simulink model "DL_wKoopman_SimulinkModel"  (R2020b)
settings: Solver=VariableStepAuto  StartTime=0.0  StopTime=10.0  RelTol=1e-3
values from neighbouring files (symbols this model uses):
  B = 0.00732    [DCMotor_Shifted.m]
  C2_new = C2_lift    [DL_wKoopman.m]
  IC_augmented = [x0' zeros(1,Nlift+Nrbf)]    [DL_wKoopman.m]
  IC_original = [x0' zeros(1,Nrbf)]    [DL_wKoopman.m]
  J = 0.00441    [DCMotor_Shifted.m]
  K = dlqr(A_new,B2_new,Q,R)    [DL_wKoopman.m]
  km = 0.253    [DCMotor_Shifted.m]
  La = 0.314    [DCMotor_Shifted.m]
  Ra = 12.345    [DCMotor_Shifted.m]
  sysKF = ss(A_new-Kf*C2_new,[B2_new Kf],eye(Nlift),0*[B2_new Kf])    [DL_wKoopman.m]
  taul = 1.47    [DCMotor_Shifted.m]
  ua = 60    [DCMotor_Shifted.m]
  x0 = [5;30]    [DL_wKoopman.m]
undefined symbols (not defined in the file or in its folder): K_hinf_aug
libraries: simulink x1
settings Model: Creator=anujpal  LastModifiedBy=anujpal

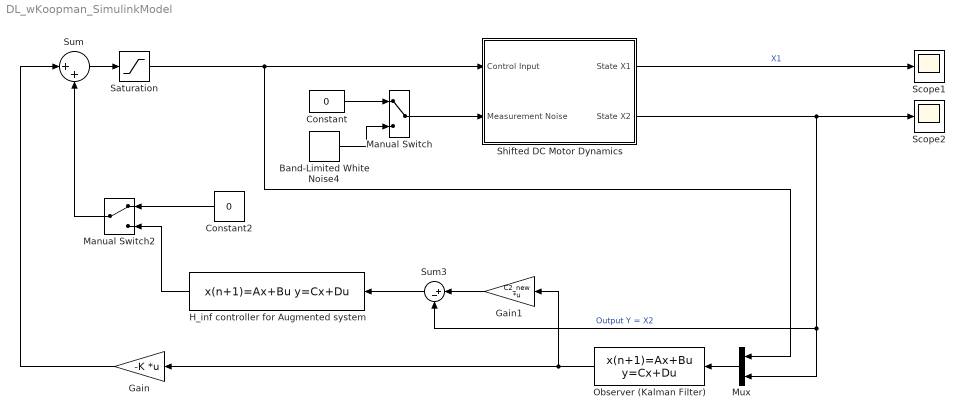
== system DL_wKoopman_SimulinkModel ==
  Band-Limited White Noise4 : simulink/Sources/Band-Limited White Noise  Cov=1  Ts=0.01  seed=245
  Constant : Constant  Value=0
  Constant2 : Constant  Value=0
  Gain : Gain  Gain=-K  Multiplication=Matrix(K*u) (u vector)
  Gain1 : Gain  Gain=C2_new  Multiplication=Matrix(K*u) (u vector)
  H_inf controller for Augmented system : DiscreteStateSpace  A=K_hinf_aug.A  B=K_hinf_aug.B  C=K_hinf_aug.C  D=K_hinf_aug.D  InitialCondition=IC_augmented  SampleTime=-1
  Manual Switch : ManualSwitch
  Manual Switch2 : ManualSwitch
  Mux : Mux  Inputs=2
  Observer (Kalman Filter) : DiscreteStateSpace  A=sysKF.A  B=sysKF.B  C=sysKF.C  D=sysKF.D  InitialCondition=IC_original  SampleTime=-1
  Saturation : Saturate  UpperLimit=4  LowerLimit=-4
  Scope1 : Scope
  Scope2 : Scope
  Shifted DC Motor Dynamics : Subsystem
  Sum : Sum  Inputs=|++
  Sum3 : Sum  Inputs=|+-
  wires:
  Shifted DC Motor Dynamics/2(State X2) -> Scope2/1, Mux/2, Sum3/2  "Output Y = X2"
  Manual Switch/1 -> Shifted DC Motor Dynamics/2(Measurement Noise)
  Shifted DC Motor Dynamics/1(State X1) -> Scope1/1  "X1"
  Sum3/1 -> H_inf controller for Augmented system/1
  Observer (Kalman Filter)/1 -> Gain/1, Gain1/1
  Sum/1 -> Saturation/1
  Constant/1 -> Manual Switch/1
  Mux/1 -> Observer (Kalman Filter)/1
  Constant2/1 -> Manual Switch2/1
  Manual Switch2/1 -> Sum/2
  H_inf controller for Augmented system/1 -> Manual Switch2/2
  Gain/1 -> Sum/1
  Band-Limited White Noise4/1 -> Manual Switch/2
  Gain1/1 -> Sum3/1
  Saturation/1 -> Shifted DC Motor Dynamics/1(Control Input), Mux/1

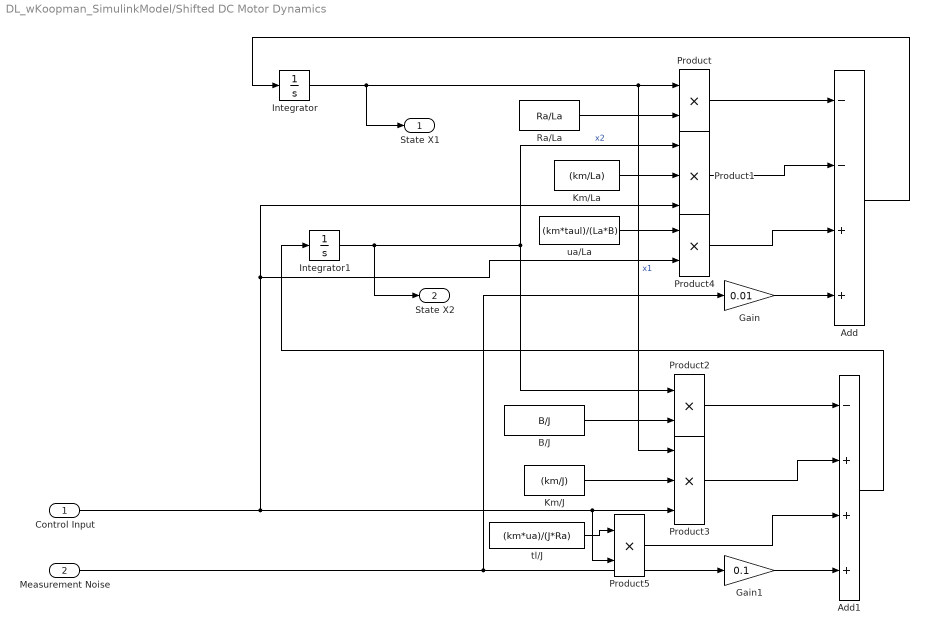
== system DL_wKoopman_SimulinkModel/Shifted DC Motor Dynamics ==
  Control Input : Inport
  Measurement Noise : Inport  Port=2
  Add : Sum  Inputs=--++
  Add1 : Sum  Inputs=-+++
  B/J : Constant  Value=B/J
  Gain : Gain  Gain=0.01
  Gain1 : Gain  Gain=0.1
  Integrator : Integrator  InitialCondition=x0(1)
  Integrator1 : Integrator  InitialCondition=x0(2)
  Km/J : Constant  Value=(km/J)
  Km/La : Constant  Value=(km/La)
  Product{,2,4..5} (4 alike) : Product
  Product1 : Product  Inputs=3
  Product3 : Product  Inputs=3
  Ra/La : Constant  Value=Ra/La
  tl/J : Constant  Value=(km*ua)/(J*Ra)
  ua/La : Constant  Value=(km*taul)/(La*B)
  State X1 : Outport
  State X2 : Outport  Port=2
  wires:
  Product5/1 -> Add1/3
  tl/J/1 -> Product5/1
  ua/La/1 -> Product4/1
  Product4/1 -> Add/3
  Measurement Noise/1 -> Gain1/1, Gain/1
  Gain1/1 -> Add1/4
  Gain/1 -> Add/4
  Integrator/1 -> State X1/1, Product/1, Product3/1  "x1"
  Product/1 -> Add/1
  Control Input/1 -> Product5/2, Product3/3, Product1/3, Product4/2
  Integrator1/1 -> State X2/1, Product1/1, Product2/1  "x2"
  Product1/1 -> Add/2
  Add/1 -> Integrator/1
  Ra/La/1 -> Product/2
  Add1/1 -> Integrator1/1
  Product3/1 -> Add1/2
  Km/J/1 -> Product3/2
  Product2/1 -> Add1/1
  B/J/1 -> Product2/2
  Km/La/1 -> Product1/2
